simulink subsystem "stateMachine"  (R2022b)
settings: Solver=VariableStepAuto  StartTime=0.0  StopTime=10.0  RelTol=1e-3
libraries: Raptor_lib x2
settings Model: Creator=serga  LastModifiedBy=serga

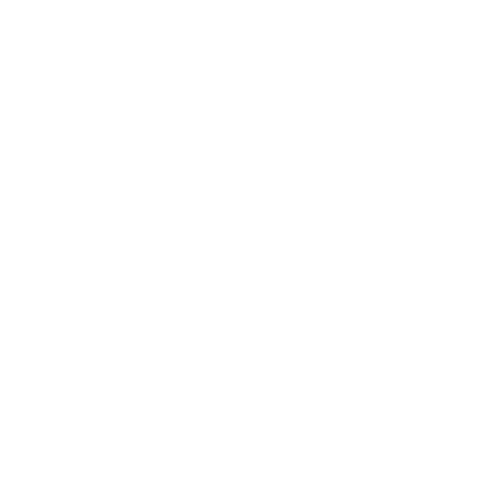
[thumbnail: Simulink's stored preview of the top-level diagram]
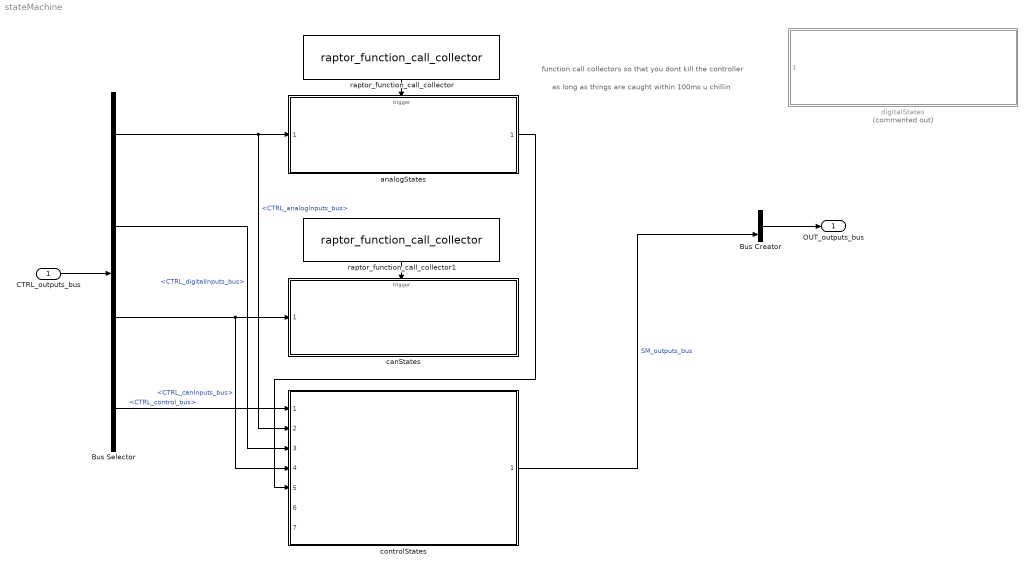
== system stateMachine ==
  note: as long as things are caught within 100ms u chillin
  note: function call collectors so that you dont kill the controller
  CTRL_outputs_bus : Inport
  Bus Creator : BusCreator  Inputs=2
  Bus Selector : BusSelector  OutputSignals=CTRL_analogInputs_bus,CTRL_digitalInputs_bus,CTRL_canInputs_bus,CTRL_control_bus
  analogStates : Subsystem  ReferencedSubsystem=analogStates
  canStates : Subsystem  ReferencedSubsystem=canStates
  controlStates : Subsystem  ReferencedSubsystem=controlStates
  digitalStates : Subsystem  Commented=on  ReferencedSubsystem=digitalStates
  raptor_function_call_collector : Raptor_lib/Triggers/raptor_function_call_collector  count=8
      settings: SourceProductName=Raptor
  raptor_function_call_collector1 : Raptor_lib/Triggers/raptor_function_call_collector  count=8
      settings: SourceProductName=Raptor
  OUT_outputs_bus : Outport
  wires:
  CTRL_outputs_bus/1 -> Bus Selector/1
  Bus Selector/4 -> controlStates/1  "<CTRL_control_bus>"
  Bus Selector/3 -> canStates/1, controlStates/4  "<CTRL_canInputs_bus>"
  Bus Selector/2 -> controlStates/3  "<CTRL_digitalInputs_bus>"
  Bus Selector/1 -> analogStates/1, controlStates/2  "<CTRL_analogInputs_bus>"
  analogStates/1 -> controlStates/5
  ? -> controlStates/6
  ? -> controlStates/7
  controlStates/1 -> Bus Creator/2  "SM_outputs_bus"
  Bus Creator/1 -> OUT_outputs_bus/1
  raptor_function_call_collector/1 -> analogStates/Trigger
  raptor_function_call_collector1/1 -> canStates/Trigger
